simulink model "Cart_Inverted_Pendulum"  (R2018b)
settings: Solver=VariableStepAuto  StartTime=0.0  StopTime=50  RelTol=1e-3
undefined symbols (not defined in the file or in its folder): sigbuilder_block
settings Model: Creator=daiba  LastModifiedBy=daiba

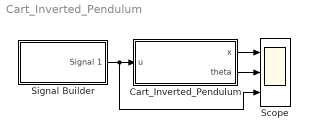
== system Cart_Inverted_Pendulum ==
  Cart_Inverted_Pendulum : Subsystem  mask{MM=1.2, m=0.2, l=1.3, g=9.81, b_1=0.2, b_2=0.15, theta_zero=-pi/18, x_zero=0}
      mask prompts: MM "Khoi luong cua xe (kg)"; m "Khoi luong cua con lac (kg)"; l "Chieu dai cua con lac (m)"; g "Gia toc trong truong (m/s2)"; b_1 "He so ma sat b1"; b_2 "He so ma sat b2"; theta_zero "Goc lech theta ban dau"; x_zero "Vi tri xe ban dau"
  Scope : Scope  NumInputPorts=3
  Signal Builder : Subsystem  Tag=STV Subsys  LoadFcn=sigbuilder_block('load',[411.6 3 546.6 453 ]);  StartFcn=sigbuilder_block('start');  StopFcn=sigbuilder_block('stop');  ClipboardFcn=sigbuilder_block('clipboard');  mask(Sigbuilder block){tuvar=[0:10]}
      mask help: Simulink:masks:SigbuilderBlock_MD
      mask init:
      | if ~strcmp(get_param(bdroot(gcbh),'SimulationStatus'),'stopped') tuvar = sigbuilder_block('maskInit'); end
      settings: CopyFcn=sigbuilder_block('copy');  DeleteFcn=sigbuilder_block('delete');  ModelCloseFcn=sigbuilder_block('modelClose');  PreSaveFcn=sigbuilder_block('preSave');  PauseFcn=sigbuilder_block('pause');  ContinueFcn=sigbuilder_block('continue');  NameChangeFcn=sigbuilder_block('namechange');  OpenFcn=sigbuilder_block('open',[437.6 199.2 550.4 400 ]);  CloseFcn=sigbuilder_block('close');
      mask Display: plot(0, 0, 100, 100,[2, 2, 32, 32, 2], [68, 8, 8, 68, 68],[32, 2], [38, 38], [32, 19, 2],[53, 60, 44], [32, 17, 17, 2],[16, 16, 31, 31]);txt = getActiveGroup(gcbh);text(2, 100, txt,'verticalAlignment', 'top');
  wires:
  Signal Builder/1(Signal 1) -> Scope/3, Cart_Inverted_Pendulum/1(u)
  Cart_Inverted_Pendulum/1(x) -> Scope/1
  Cart_Inverted_Pendulum/2(theta) -> Scope/2

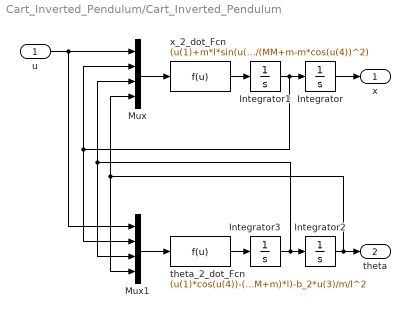
== system Cart_Inverted_Pendulum/Cart_Inverted_Pendulum ==
  u : Inport
  Integrator : Integrator  InitialCondition=x_zero
  Integrator1 : Integrator
  Integrator2 : Integrator  InitialCondition=theta_zero
  Integrator3 : Integrator
  Mux : Mux
  Mux1 : Mux
  theta_2_dot_Fcn : Fcn  Expr=(u(1)*cos(u(4))-(MM+m)*g*sin(u(4))+m*l*cos(u(4))*sin(u(4))*u(3)^2+b_2/l*u(3)*cos(u(4))^2-b_1*u(2)*cos(u(4)))/(m*l*cos(u(4))^2-(MM+m)*l)-b_2*u(3)/m/l^2
  x_2_dot_Fcn : Fcn  Expr=(u(1)+m*l*sin(u(4))*u(3)^2-m*g*cos(u(4))*sin(u(4))+b_2/l*u(3)*cos(u(4))-b_1*u(2))/(MM+m-m*cos(u(4))^2)
  x : Outport
  theta : Outport  Port=2
  wires:
  Integrator/1 -> x/1
  x_2_dot_Fcn/1 -> Integrator1/1
  theta_2_dot_Fcn/1 -> Integrator3/1
  Mux/1 -> x_2_dot_Fcn/1
  Mux1/1 -> theta_2_dot_Fcn/1
  u/1 -> Mux1/1, Mux/1
  Integrator1/1 -> Mux1/2, Mux/2, Integrator/1
  Integrator3/1 -> Mux1/3, Mux/3, Integrator2/1
  Integrator2/1 -> Mux1/4, Mux/4, theta/1

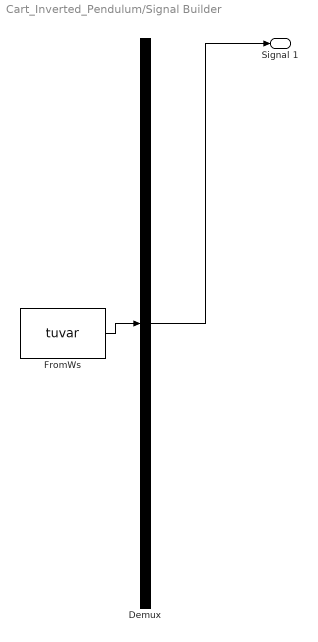
== system Cart_Inverted_Pendulum/Signal Builder ==
  Demux : Demux  Tag=STV Demux  Outputs=1
  FromWs : FromWorkspace  Tag=STV FromWs  VariableName=tuvar  SampleTime=0
      SigBuilderData=|
      | common.afterFinalStr = 'Extrapolate'
      | common.sampleTime = 0
      | dataSet.timeRange = [0 10]
      | dataSet.name = 'Group 1'
      | sbobj.Groups.Name = 'Group 1'
      | sbobj.Groups.Signals.Name = 'Signal 1'
      | sbobj.Groups.Signals.XData = [0 4 6 10]
      | sbobj.Groups.Signals.YData = [0 0 0 0]
  Signal 1 : Outport  Tag=STV Outport
  wires:
  Demux/1 -> Signal 1/1
  FromWs/1 -> Demux/1
